simulink model "ikinci_dosya"  (R2018a)
settings: Solver=VariableStepAuto  StartTime=0.0  StopTime=10.0  RelTol=1e-3
settings Model: Creator=PC_393_ADMIN  LastModifiedBy=PC_393_ADMIN

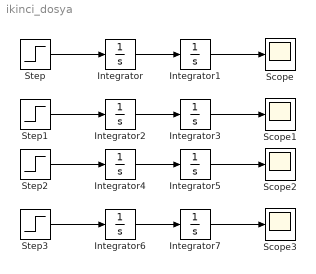
== system ikinci_dosya ==
  Integrator{,1..7} (8 alike) : Integrator
  Scope{,1..3} (4 alike) : Scope
  Step{,1..3} (4 alike) : Step  SampleTime=0
  wires:
  Integrator1/1 -> Scope/1
  Step/1 -> Integrator/1
  Integrator/1 -> Integrator1/1
  Integrator2/1 -> Integrator3/1
  Step1/1 -> Integrator2/1
  Integrator3/1 -> Scope1/1
  Integrator7/1 -> Scope3/1
  Step3/1 -> Integrator6/1
  Integrator6/1 -> Integrator7/1
  Integrator4/1 -> Integrator5/1
  Step2/1 -> Integrator4/1
  Integrator5/1 -> Scope2/1
